simulink model "CicDecimator75"  (Simulink 6.3)
settings: Solver=VariableStepDiscrete  SolverMode=SingleTasking  StartTime=0  StopTime=7000  FixedStep=1  RelTol=1e-3
InitFcn:
  | %% DSPBuilder Start
  | alt_dspbuilder_update_model(bdroot)
  | %% DSPBuilder End
libraries: allblocks_alteradspbuilder2 x15
settings Model: Creator=mjervis  LastModifiedBy=LKONG
settings DataIOCC: SignalLoggingName=sigsOut
settings OptimizationCC: BooleanDataType=off  InlineInvariantSignals=on
settings DebuggingCC: SolverPrmCheckMsg=none
settings HardwareCC: TargetUnknown=on

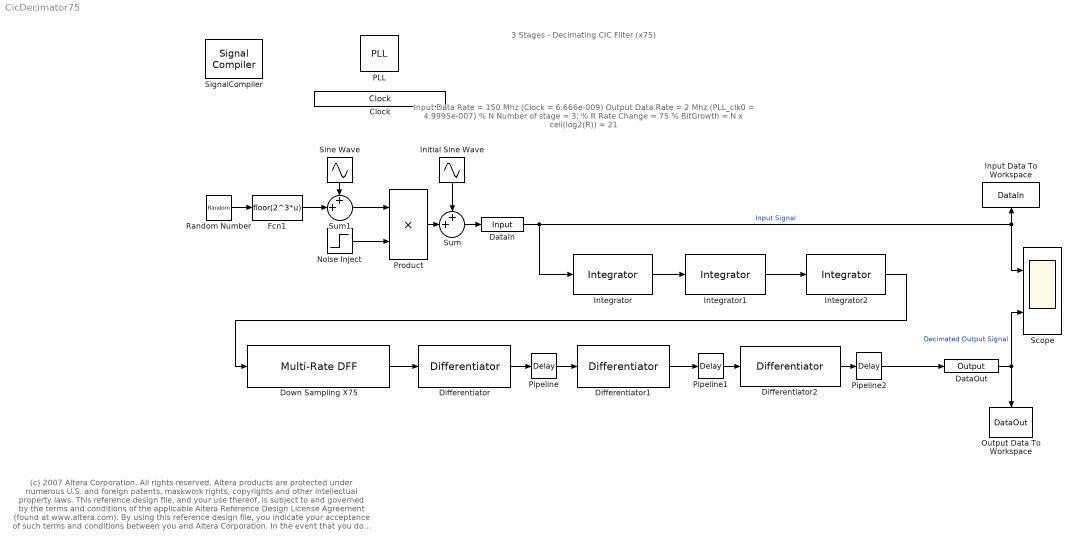
== system CicDecimator75 ==
  note: 3 Stages - Decimating CIC Filter (x75)
  note: (c) 2007 Altera Corporation. All rights reserved.  Altera products are protected under numerous U.S. and foreign patents, maskwork rights, copyrights and other intellectual property laws.
      | This reference design file, and your use thereof, is subject to and governed by the terms and conditions of the applicable Altera Reference Design License Agreement (found at www.altera.com).
      | By using this reference design file, you indicate your acceptance of such terms and conditions between you and Altera Corporation.
      | In the event that you do not agree with such terms and conditions, you may not use the reference design file and please promptly destroy any copies you have made.
      | This reference design file being provided on an "as-is" basis and as an accommodation and therefore all warranties, representations or guarantees of any kind (whether express, implied or statutory)
      | including, without limitation, warranties of merchantability, non-infringement, or fitness for a particular purpose, are specifically disclaimed.
      | By making this reference design file available, Altera expressly does not recommend, suggest or require that this reference design file be used in combination with any other product not provided by Altera
  note: Input Data Rate    = 150 Mhz (Clock       = 6.666e-009)
      | Output Data Rate = 2 Mhz     (PLL_clk0 = 4.9995e-007)
      |
      | % N Number of stage = 3,
      | % R Rate Change      = 75
      | % BitGrowth               = N x ceil(log2(R)) =  21
  Clock : allblocks_alteradspbuilder2/Clock  ClockPeriod=20/3  ClockPeriodUnit=ns  SampleTime=1  SimulationStartCycle=5  PhaseOffset=0  Reset=aclr  ResetType=Active Low  Export=off
  DataIn : allblocks_alteradspbuilder2/Input  iofile=d:\wsTrunk\workspace\Documentation\DesignExamples\Demos\Filters\CicFilter\Decimator\tb_CicDecimator75\CicDecimator75_DataIn.salt  BusType=Signed Integer  bwl=8  bwr=0  SpecifyClock=off  clock=Clock  PORTTYPE=Input
  DataOut : allblocks_alteradspbuilder2/Output  iofile=d:\wsTrunk\workspace\Documentation\DesignExamples\Demos\Filters\CicFilter\Decimator\tb_CicDecimator75\CicDecimator75_DataOut.capture  BusType=Signed Integer  bwl=29  bwr=0  PORTTYPE=Output
  Differentiator : allblocks_alteradspbuilder2/Differentiator  bwl=29  depth=1  use_ena=off  use_sclr=off
  Differentiator1 : allblocks_alteradspbuilder2/Differentiator  bwl=29  depth=1  use_ena=off  use_sclr=off
  Differentiator2 : allblocks_alteradspbuilder2/Differentiator  bwl=29  depth=1  use_ena=off  use_sclr=off
  Down Sampling X75 : allblocks_alteradspbuilder2/Multi-Rate DFF  pipeline=1  UseBaseClock=off  clock=PLL_clk0  use_ena=off  use_sclr=off
  Fcn1 : Fcn  Expr=floor(2^3*u)
  Initial Sine Wave : Sin  Orientation=down  SineType=Sample based  Amplitude=2^6 -1  Samples=1000  SampleTime=1
  Input Data To Workspace : ToWorkspace  VariableName=DataIn  SampleTime=-1  SaveFormat=Array
      settings: Orientation=up
  Integrator : allblocks_alteradspbuilder2/Integrator  bwl=29  depth=1  use_ena=off  use_sclr=off
  Integrator1 : allblocks_alteradspbuilder2/Integrator  bwl=29  depth=1  use_ena=off  use_sclr=off
  Integrator2 : allblocks_alteradspbuilder2/Integrator  bwl=29  depth=1  use_ena=off  use_sclr=off
  Noise Inject : Step  Time=2500  SampleTime=1
  Output Data To Workspace : ToWorkspace  VariableName=DataOut  SampleTime=-1  SaveFormat=Array
      settings: Orientation=down
  PLL : allblocks_alteradspbuilder2/PLL  clock_mult=[75, 75, 3, 4, 1, 1, 1, 1, 1]  clock_divide=[1, 1, 3, 1, 1, 1, 1, 1, 1]  clock_export=[0, 0, 0, 0, 0, 0, 0, 0, 0]  num_clocks=1  input_clock=Clock  use_base_clock=on
  Pipeline : allblocks_alteradspbuilder2/Delay  pipeline=1  ClockPhase=1  use_ena=off  use_sclr=off  use_init=off  reset_value=1
  Pipeline1 : allblocks_alteradspbuilder2/Delay  pipeline=1  ClockPhase=1  use_ena=off  use_sclr=off  use_init=off  reset_value=1
  Pipeline2 : allblocks_alteradspbuilder2/Delay  pipeline=1  ClockPhase=1  use_ena=off  use_sclr=off  use_init=off  reset_value=1
  Product : Product  SaturateOnIntegerOverflow=on  InputSameDT=on
  Random Number : RandomNumber  Variance=8  SampleTime=1
  Scope : Scope  NumInputPorts=2
      settings: TimeRange=7000  YMin=-150~-30000000  YMax=150~30000000  MaxDataPoints=10000
  SignalCompiler : allblocks_alteradspbuilder2/Signal Compiler  DeviceFamily=Stratix III  DeviceName=AUTO  EnableSignalTap=off  SignalTapDepth=128  UseBoardBlock=off  StpUseDefaultClock=on  StpClock=clock
  Sine Wave : Sin  Orientation=down  SineType=Sample based  Amplitude=2^3 -1  Samples=500  SampleTime=1
  Sum : Sum  Inputs=++|  SaturateOnIntegerOverflow=on  InputSameDT=on
  Sum1 : Sum  Inputs=++|  SaturateOnIntegerOverflow=on  InputSameDT=on
  wires:
  Random Number/1 -> Fcn1/1
  Differentiator/1 -> Pipeline/1
  Integrator/1 -> Integrator1/1
  Differentiator1/1 -> Pipeline1/1
  Integrator1/1 -> Integrator2/1
  Sum/1 -> DataIn/1
  Noise Inject/1 -> Product/2
  Sum1/1 -> Product/1
  DataOut/1 -> Scope/2, Output Data To Workspace/1  "Decimated Output Signal"
  Differentiator2/1 -> Pipeline2/1
  DataIn/1 -> Integrator/1, Scope/1, Input Data To Workspace/1  "Input Signal"
  Down Sampling X75/1 -> Differentiator/1
  Integrator2/1 -> Down Sampling X75/1
  Pipeline/1 -> Differentiator1/1
  Pipeline1/1 -> Differentiator2/1
  Pipeline2/1 -> DataOut/1
  Fcn1/1 -> Sum1/2
  Sine Wave/1 -> Sum1/1
  Product/1 -> Sum/2
  Initial Sine Wave/1 -> Sum/1
